simulink model "XbeeSerialRead"  (R2014a)
settings: Solver=ode3  SolverMode=SingleTasking  StartTime=0.0  StopTime=10.0  RelTol=1e-3
libraries: arduinolib x3
settings Model: ExtModeTrigDuration=2  Creator=beaverl  LastModifiedBy=beaverl
settings OptimizationCC: OptimizeModelRefInitCode=on  LifeSpan=1
settings DebuggingCC: UnderspecifiedInitializationDetection=Classic  SolverPrmCheckMsg=none
settings HardwareCC: ProdBitPerInt=16  ProdBitPerPointer=8  ProdIntDivRoundTo=Zero  ProdEndianess=LittleEndian  ProdWordSize=8  ProdHWDeviceType=Atmel->AVR
settings RTWCC: SystemTargetFile=realtime.tlc  GenerateMakefile=off  TemplateMakefile=realtime.tmf  Description=Run on Target Hardware  RTWVerbose=off  ProcessScript=realtime_make_rtw_hook
settings STFCustomTargetCC: TargetLibSuffix=.a  GenerateSampleERTMain=on  ConcurrentExecutionCompliant=off  GeneratePreprocessorConditionals=Use local settings  ERTCustomFileBanners=on  SupportNonInlinedSFcns=off  SupportVariableSizeSignals=on  MATLABClassNameForMDSCustomization=Simulink.SoftwareTarget.ERTCustomization  GRTInterface=off  SystemTargetFile=realtime.tlc
settings ERTTargetCC: CombineOutputUpdateFcns=off  SupportContinuousTime=on  SupportVariableSizeSignals=on  ExtModeTransport=3  ExtModeMexFile=ext_serial_win32_comm  ExtModeMexArgs=0 1 9600  ERTSrcFileBannerTemplate=realtime_code_template.cgt  ERTHdrFileBannerTemplate=realtime_code_template.cgt  ERTDataSrcFileTemplate=realtime_code_template.cgt  ERTDataHdrFileTemplate=realtime_code_template.cgt  ERTCustomFileTemplate=realtime_file_process.tlc

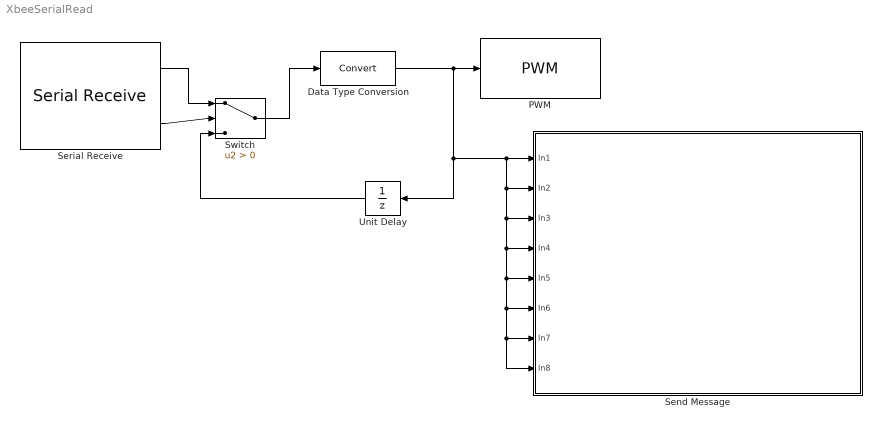
== system XbeeSerialRead ==
  Data Type Conversion : DataTypeConversion  SaturateOnIntegerOverflow=on
  PWM : arduinolib/PWM  pinNumber=5
  Send Message : Subsystem
  Serial Receive : arduinolib/Serial Receive  portNumber=1  showOutStatus=on  sampleTime=0.02
  Switch : Switch  Criteria=u2 > Threshold
  Unit Delay : UnitDelay  SampleTime=-1
  wires:
  Data Type Conversion/1 -> Unit Delay/1, Send Message/8(In8), Send Message/7(In7), Send Message/6(In6), Send Message/5(In5), Send Message/4(In4), Send Message/3(In3), Send Message/2(In2), Send Message/1(In1), PWM/1
  Serial Receive/2 -> Switch/2
  Serial Receive/1 -> Switch/1
  Switch/1 -> Data Type Conversion/1
  Unit Delay/1 -> Switch/3

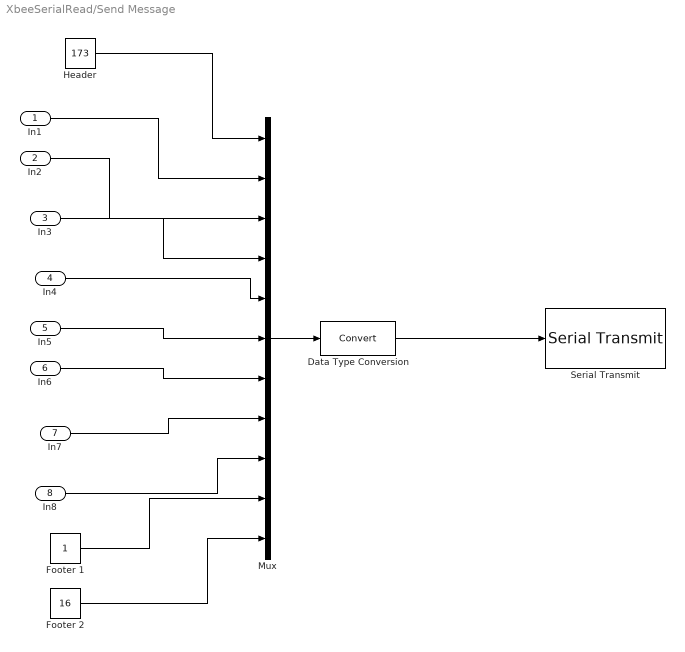
== system XbeeSerialRead/Send Message ==
  In1 : Inport
  In2 : Inport  Port=2
  In3 : Inport  Port=3
  In4 : Inport  Port=4
  In5 : Inport  Port=5
  In6 : Inport  Port=6
  In7 : Inport  Port=7
  In8 : Inport  Port=8
  Data Type Conversion : DataTypeConversion  SaturateOnIntegerOverflow=on
  Footer 1 : Constant
  Footer 2 : Constant  Value=16
  Header : Constant  Value=173
  Mux : Mux  Inputs=11
  Serial Transmit : arduinolib/Serial Transmit  portNumber=1
  wires:
  In1/1 -> Mux/2
  In2/1 -> Mux/3
  In3/1 -> Mux/4
  In4/1 -> Mux/5
  In5/1 -> Mux/6
  In6/1 -> Mux/7
  In7/1 -> Mux/8
  In8/1 -> Mux/9
  Header/1 -> Mux/1
  Footer 1/1 -> Mux/10
  Footer 2/1 -> Mux/11
  Mux/1 -> Data Type Conversion/1
  Data Type Conversion/1 -> Serial Transmit/1
